simulink model "IndicatorControl"  (R2025a)
settings: Solver=FixedStepDiscrete  StartTime=0.0  StopTime=10.0  RelTol=1e-3
settings Model: Creator=srika  LastModifiedBy=srika
settings OptimizationCC: DefaultParameterBehavior=Inlined  EnhancedBackFolding=on  PassReuseOutputArgsAs=Individual arguments  ZeroExternalMemoryAtStartup=off  ZeroInternalMemoryAtStartup=off  OptimizeBlockOrder=speed  DifferentSizesBufferReuse=on  OptimizationCustomize=off  EfficientTunableParamExpr=on
settings DebuggingCC: ParameterTunabilityLossMsg=error
settings SFSimCC: MATLABDynamicMemAlloc=off
settings RTWCC: SystemTargetFile=ert.tlc  GenCodeOnly=on  TemplateMakefile=ert_default_tmf  Description=Embedded Coder
settings CodeAppCC: ForceParamTrailComments=on  IgnoreCustomStorageClasses=off  OperatorAnnotations=on  SimulinkDataObjDesc=on  SFDataObjDesc=on  InsertBlockDesc=on
settings ERTTargetCC: ExtModeTransport=0.0  ExtModeStaticAlloc=off  ExtModeMexFile=ext_comm  ExtModeIntrfLevel=Level1  ERTCustomFileTemplate=example_file_process.tlc  TargetLangStandard=C99 (ISO)  GenerateSampleERTMain=on

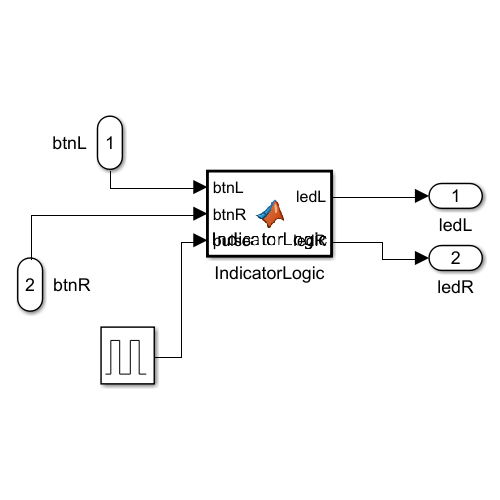
[thumbnail: Simulink's stored preview of the top-level diagram]
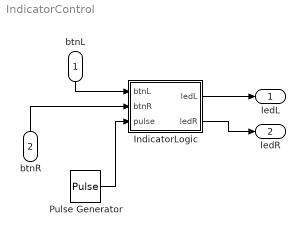
== system IndicatorControl ==
  btnL : Inport
  btnR : Inport  Port=2
  IndicatorLogic : MATLAB Function  TreatAsAtomicUnit=on
  Pulse Generator : DiscretePulseGenerator  PulseType=Time based  Period=0.6  PulseWidth=50  PhaseDelay=0.1
  ledL : Outport
  ledR : Outport  Port=2
  wires:
  btnL/1 -> IndicatorLogic/1(btnL)
  btnR/1 -> IndicatorLogic/2(btnR)
  Pulse Generator/1 -> IndicatorLogic/3(pulse)
  IndicatorLogic/1(ledL) -> ledL/1
  IndicatorLogic/2(ledR) -> ledR/1

== matlab function IndicatorControl/IndicatorLogic ==
  data: btnL input; ledL output; btnR input; pulse input; ledR output
function [ledL, ledR] = IndicatorLogic(btnL, btnR, pulse)
% Simple full logic in one block
% Inputs: btnL, btnR (boolean), pulse (toggle signal)
% Outputs: ledL, ledR (boolean)

persistent countL countR
if isempty(countL)
    countL = 0;
    countR = 0;
end

% Default outputs
ledL = 0;
ledR = 0;

% Count how long buttons are pressed
if btnL
    countL = countL + 1;
else
    countL = 0;
end

if btnR
    countR = countR + 1;
else
    countR = 0;
end

% Check if pressed ≥ 1 second (0.1s × 10 = 1s)
pressedL = (countL >= 10);
pressedR = (countR >= 10);

% Hazard logic: both buttons pressed
if pressedL && pressedR
    ledL = pulse;
    ledR = pulse;
elseif pressedL
    ledL = pulse;
    ledR = 0;
elseif pressedR
    ledR = pulse;
    ledL = 0;
end
